simulink subsystem "Impedance_Measurement_Algorithm"  (R2024b)
settings: Solver=VariableStepAuto  StartTime=0.0  StopTime=10.0  RelTol=1e-3
values from neighbouring files (symbols this model uses):
  frequencies = frequencies(frequencies >= start_freq &  frequencies <= end_freq )    [parameters.m]    (also in prepImplementationFigure.m = linspace(0.1,5000,1000000))
  num_frequencies = length(frequencies)    [parameters.m]
libraries: simulink x4, dspstat3 x2, dspsigops x2
settings Model: Creator=JesseJabezArendse  LastModifiedBy=JesseJabezArendse
settings RTWCC: GPUComputeCapability=3.5

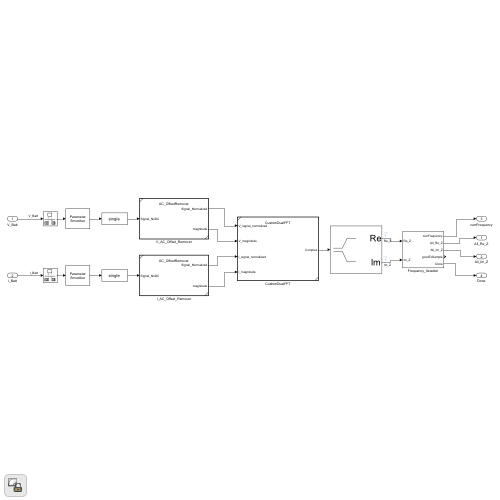
[thumbnail: Simulink's stored preview of the top-level diagram]
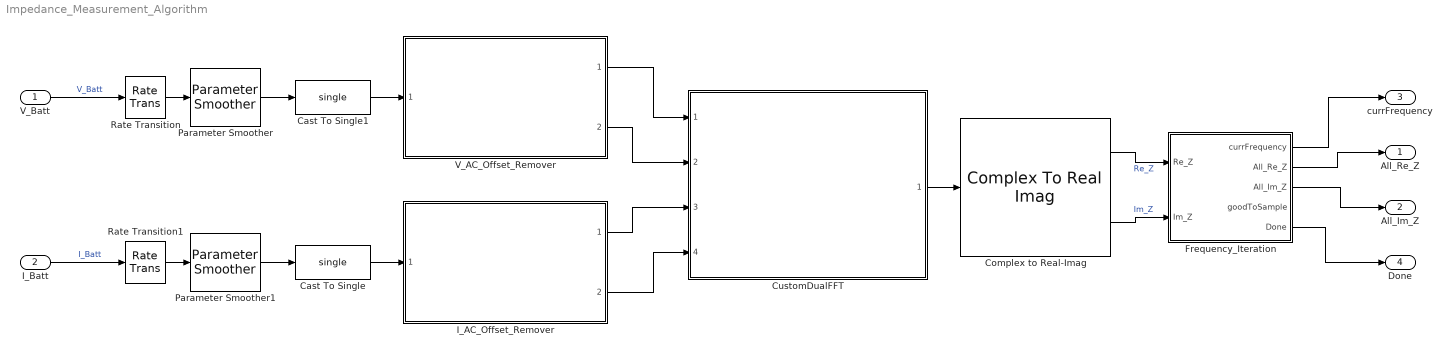
== system Impedance_Measurement_Algorithm ==
  V_Batt : Inport
  I_Batt : Inport  Port=2
  Cast To Single : DataTypeConversion  OutDataTypeStr=single  SaturateOnIntegerOverflow=off  RndMeth=Floor
  Cast To Single1 : DataTypeConversion  OutDataTypeStr=single  SaturateOnIntegerOverflow=off  RndMeth=Floor
  Complex to Real-Imag : ComplexToRealImag
  CustomDualFFT : Subsystem  TreatAsAtomicUnit=on  ReferencedSubsystem=CustomDualFFT
  Frequency_Iteration : Subsystem
  I_AC_Offset_Remover : Subsystem  TreatAsAtomicUnit=on  ReferencedSubsystem=AC_OffsetRemover
  Parameter Smoother : dspsigops/Parameter Smoother  NumParameters=1  SmoothingMode=Smoothing factor  SmoothingFactorPort=off  SmoothingFactor=0.8  SmoothingTimePort=off  SmoothingTime=1  SampleTime=-1  SimulateUsing=Code generation
  Parameter Smoother1 : dspsigops/Parameter Smoother  NumParameters=1  SmoothingMode=Smoothing factor  SmoothingFactorPort=off  SmoothingFactor=0.8  SmoothingTimePort=off  SmoothingTime=1  SampleTime=-1  SimulateUsing=Code generation
  Rate Transition : RateTransition  Integrity=off
  Rate Transition1 : RateTransition  Integrity=off
  V_AC_Offset_Remover : Subsystem  TreatAsAtomicUnit=on  ReferencedSubsystem=AC_OffsetRemover
  All_Re_Z : Outport  OutDataTypeStr=single  PortDimensions=num_frequencies
  All_Im_Z : Outport  Port=2  OutDataTypeStr=single  PortDimensions=num_frequencies
  currFrequency : Outport  Port=3  OutDataTypeStr=single  PortDimensions=1
  Done : Outport  Port=4  OutDataTypeStr=boolean  PortDimensions=1
  wires:
  CustomDualFFT/1 -> Complex to Real-Imag/1
  V_Batt/1 -> Rate Transition/1  "V_Batt"
  I_Batt/1 -> Rate Transition1/1  "I_Batt"
  I_AC_Offset_Remover/2 -> CustomDualFFT/4
  Rate Transition/1 -> Parameter Smoother/1
  Parameter Smoother/1 -> Cast To Single1/1
  Rate Transition1/1 -> Parameter Smoother1/1
  Parameter Smoother1/1 -> Cast To Single/1
  V_AC_Offset_Remover/1 -> CustomDualFFT/1
  V_AC_Offset_Remover/2 -> CustomDualFFT/2
  I_AC_Offset_Remover/1 -> CustomDualFFT/3
  Cast To Single/1 -> I_AC_Offset_Remover/1
  Cast To Single1/1 -> V_AC_Offset_Remover/1
  Complex to Real-Imag/1 -> Frequency_Iteration/1(Re_Z)  "Re_Z"
  Complex to Real-Imag/2 -> Frequency_Iteration/2(Im_Z)  "Im_Z"
  Frequency_Iteration/5(Done) -> Done/1
  Frequency_Iteration/1(currFrequency) -> currFrequency/1
  Frequency_Iteration/2(All_Re_Z) -> All_Re_Z/1
  Frequency_Iteration/3(All_Im_Z) -> All_Im_Z/1

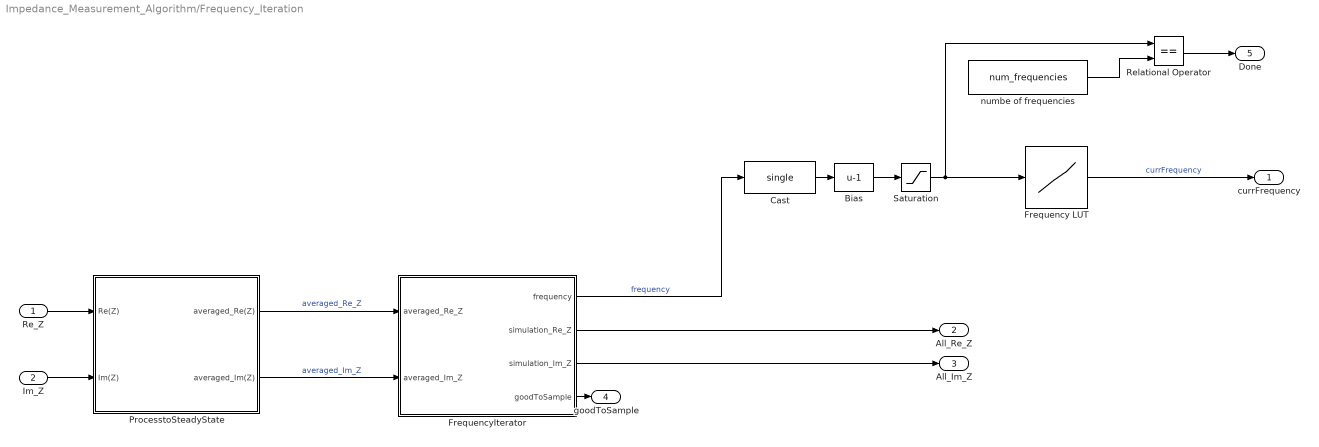
== system Impedance_Measurement_Algorithm/Frequency_Iteration ==
  Re_Z : Inport
  Im_Z : Inport  Port=2
  Bias : Bias  Bias=-1  SaturateOnIntegerOverflow=off
  Cast : DataTypeConversion  OutDataTypeStr=single  SaturateOnIntegerOverflow=off  RndMeth=Floor
  Frequency LUT : Lookup_n-D  NumberOfTableDimensions=1  BreakpointsForDimension1=[1:length(frequencies)]  BreakpointsForDimension1DataTypeStr=single  Table=frequencies  TableDataTypeStr=single  IntermediateResultsDataTypeStr=single  ExtrapMethod=Clip  InternalRulePriority=Speed  OutDataTypeStr=single  RndMeth=Simplest  FractionDataTypeStr=single
  FrequencyIterator : Stateflow chart  TreatAsAtomicUnit=on
      settings: PortSchema="{\"entries\":[{\"content\":{\"sides\":[{\"content\":{\"connectorIds\":[\"In1\",\"In2\"]},\"type\":\"ConnectorPlacement.EquallySpacedRectSide\",\"uuid\":\"8a288858-315b-4c22-be58-8f66fdbadcaa\"},{\"content\":{\"connectorIds\":[\"Out2\",\"Out4\",\"Out3\",\"Out1\"],\"side\":\"RIGHT\"},\"type\":\"ConnectorPlacement.EquallySpacedRectSide\",\"uuid\":\"82a50930-f4d0-4fa8-89d1-0fd36925fc15\"},{\"content\":{\"side\":\"TOP\"},\"type\":\"ConnectorPlacement.EquallySpacedRectSide\",\"uuid\":\"fce5baf5-6ef5-438e-9f22-4b36439d2679\"},{\"content\":{\"side\":\"BOTTOM\"},\"type\":\"ConnectorPlacement.EquallySpacedRectSide\",\"uuid\":\"49cb1ff5-4212-425e-a81b-a302905a2225\"}]},\"type\":\"ConnectorPlacement.EquallySpacedConnector\",\"uuid\":\"e215f3f3-8aeb-4c79-afac-af2a9039992f\"}],\"packageUris\":[\"http://schema.mathworks.com/mf0/Connector/R2020b\"],\"version\":\"1.0\"}"
  ProcesstoSteadyState : Subsystem  TreatAsAtomicUnit=on
  Relational Operator : RelationalOperator  Operator===  OutDataTypeStr=boolean  RndMeth=Simplest  InputSameDT=off
  Saturation : Saturate  UpperLimit=num_frequencies  LowerLimit=0
  numbe of frequencies : Constant  Value=num_frequencies  OutDataTypeStr=uint16  SampleTime=-1
  currFrequency : Outport  OutDataTypeStr=single  PortDimensions=1
  All_Re_Z : Outport  Port=2  OutDataTypeStr=single  PortDimensions=num_frequencies
  All_Im_Z : Outport  Port=3  OutDataTypeStr=single  PortDimensions=num_frequencies
  goodToSample : Outport  Port=4
  Done : Outport  Port=5  OutDataTypeStr=boolean  PortDimensions=1
  wires:
  Re_Z/1 -> ProcesstoSteadyState/1(Re(Z))
  Im_Z/1 -> ProcesstoSteadyState/2(Im(Z))
  FrequencyIterator/1(goodToSample) -> goodToSample/1
  FrequencyIterator/3(simulation_Im_Z) -> All_Im_Z/1
  Cast/1 -> Bias/1
  FrequencyIterator/4(simulation_Re_Z) -> All_Re_Z/1
  Frequency LUT/1 -> currFrequency/1  "currFrequency"
  Bias/1 -> Saturation/1
  numbe of frequencies/1 -> Relational Operator/2
  Relational Operator/1 -> Done/1
  FrequencyIterator/2(frequency) -> Cast/1  "frequency"
  ProcesstoSteadyState/2(averaged_Im(Z)) -> FrequencyIterator/2(averaged_Im_Z)  "averaged_Im_Z"
  Saturation/1 -> Frequency LUT/1, Relational Operator/1
  ProcesstoSteadyState/1(averaged_Re(Z)) -> FrequencyIterator/1(averaged_Re_Z)  "averaged_Re_Z"

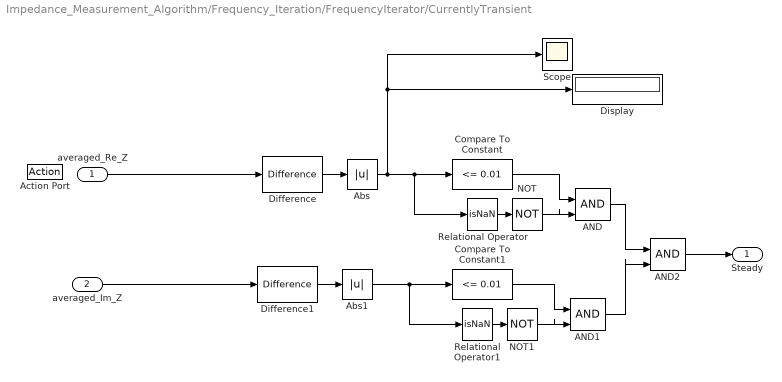
== system Impedance_Measurement_Algorithm/Frequency_Iteration/FrequencyIterator/CurrentlyTransient ==
  averaged_Re_Z : Inport
  averaged_Im_Z : Inport  Port=2
  Action Port : ActionPort
      settings: CopyFcn=Stateflow.SLINSF.SimulinkMan.removeBlockPreDeleteFcn  PreDeleteFcn=Stateflow.SLINSF.SimulinkMan.unsafePredeleteFcn
  AND : Logic  IconShape=distinctive  AllPortsSameDT=off  OutDataTypeStr=boolean
  AND1 : Logic  IconShape=distinctive  AllPortsSameDT=off  OutDataTypeStr=boolean
  AND2 : Logic  IconShape=distinctive  AllPortsSameDT=off  OutDataTypeStr=boolean
  Abs : Abs  SaturateOnIntegerOverflow=off
  Abs1 : Abs  SaturateOnIntegerOverflow=off
  Compare To Constant : simulink/Logic and Bit Operations/Compare To Constant  relop=<=  const=0.01  OutDataTypeStr=boolean
  Compare To Constant1 : simulink/Logic and Bit Operations/Compare To Constant  relop=<=  const=0.01  OutDataTypeStr=boolean
  Difference : simulink/Discrete/Difference  ICPrevInput=1  OutMin=[]  OutMax=[]  OutDataType=fixdt(1, 16)  OutScaling=2^-10  DoSatur=off
  Difference1 : simulink/Discrete/Difference  ICPrevInput=1  OutMin=[]  OutMax=[]  OutDataType=fixdt(1, 16)  OutScaling=2^-10  DoSatur=off
  Display : Display
  NOT : Logic  Operator=NOT  IconShape=distinctive  AllPortsSameDT=off  OutDataTypeStr=boolean
  NOT1 : Logic  Operator=NOT  IconShape=distinctive  AllPortsSameDT=off  OutDataTypeStr=boolean
  Relational Operator : RelationalOperator  Operator=isNaN  OutDataTypeStr=boolean  RndMeth=Simplest  InputSameDT=off
  Relational Operator1 : RelationalOperator  Operator=isNaN  OutDataTypeStr=boolean  RndMeth=Simplest  InputSameDT=off
  Scope : Scope
  Steady : Outport
  wires:
  AND2/1 -> Steady/1
  AND1/1 -> AND2/2
  AND/1 -> AND2/1
  Difference1/1 -> Abs1/1
  averaged_Im_Z/1 -> Difference1/1
  NOT1/1 -> AND1/2
  Compare To Constant1/1 -> AND1/1
  Relational Operator1/1 -> NOT1/1
  Abs1/1 -> Compare To Constant1/1, Relational Operator1/1
  NOT/1 -> AND/2
  Relational Operator/1 -> NOT/1
  Abs/1 -> Compare To Constant/1, Relational Operator/1, Display/1, Scope/1
  Compare To Constant/1 -> AND/1
  Difference/1 -> Abs/1
  averaged_Re_Z/1 -> Difference/1

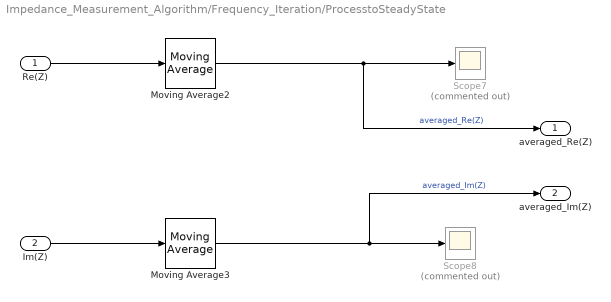
== system Impedance_Measurement_Algorithm/Frequency_Iteration/ProcesstoSteadyState ==
  Re(Z) : Inport  OutDataTypeStr=single
  Im(Z) : Inport  Port=2  OutDataTypeStr=single
  Moving Average2 : dspstat3/Moving Average  Method=Sliding window  ForgettingFactorPort=off  SpecifyWindowLength=on  WindowLength=4  OverlapLength=3  AllowArbitraryInputLength=off  ForgettingFactor=0.9  SimulateUsing=Code generation
  Moving Average3 : dspstat3/Moving Average  Method=Sliding window  ForgettingFactorPort=off  SpecifyWindowLength=on  WindowLength=4  OverlapLength=3  AllowArbitraryInputLength=off  ForgettingFactor=0.9  SimulateUsing=Code generation
  Scope7 : Scope  Commented=on
  Scope8 : Scope  Commented=on
  averaged_Re(Z) : Outport  OutDataTypeStr=single
  averaged_Im(Z) : Outport  Port=2  OutDataTypeStr=single
  wires:
  Re(Z)/1 -> Moving Average2/1
  Moving Average3/1 -> Scope8/1, averaged_Im(Z)/1  "averaged_Im(Z)"
  Moving Average2/1 -> Scope7/1, averaged_Re(Z)/1  "averaged_Re(Z)"
  Im(Z)/1 -> Moving Average3/1

== stateflow chart Impedance_Measurement_Algorithm/Frequency_Iteration/FrequencyIterator ==
  settings: updateMethod=DISCRETE  executeAtInitialization=1
  state ToTheNextFrequency
    entry:
    frequency = lastFrequency + 1;
  state WaitingForTransient
    entry:
    goodToSample = true;
    frequency = lastFrequency + 1;
  state reachedSteadyState
    entry:
    if frequency <= num_frequencies
    lastFrequency = frequency;
    simulation_Re_Z(frequency) = averaged_Re_Z;
    simulation_Im_Z(frequency) = averaged_Im_Z;
    end
    frequency = 0;
    goodToSample = false;
  state CurrentlyTransient [commented out]
  ToTheNextFrequency -> WaitingForTransient : after(0.5,sec)
  reachedSteadyState -> ToTheNextFrequency : after(0.5,sec)
  (default) -> WaitingForTransient
  WaitingForTransient -> reachedSteadyState : [after(1,sec)]
  data: sf_internal_action_state_placeholder_data local double size=1 =0; goodToSample output boolean size=1 =true; frequency output uint16 size=1 =0; averaged_Re_Z input single size=1; averaged_Im_Z input single size=1; lastFrequency local uint16 size=1 =0; simulation_Im_Z output single size=num_frequencies =zeros(num_frequencies,1); simulation_Re_Z output single size=num_frequencies =zeros(num_frequencies,1); num_frequencies local =num_frequencies
